simulink model "simulink_scheme_filter"  (R2016b)
settings: Solver=FixedStepAuto  StartTime=0.0  StopTime=20  FixedStep=0.001  RelTol=1e-3
libraries: simulink x1
settings Model: Creator=ram  LastModifiedBy=ram

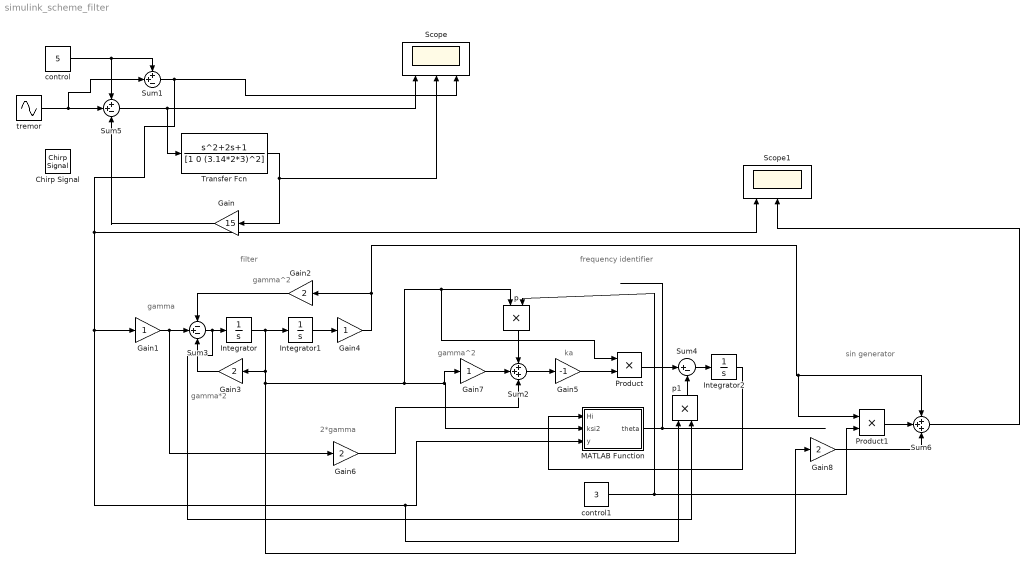
== system simulink_scheme_filter ==
  note: filter
  note: gamma
  note: gamma^2
  note: gamma*2
  note: frequency identifier
  note: ka
  note: 2*gamma
  note: gamma^2
  note: sin generator
  Chirp Signal : simulink/Sources/Chirp Signal  f1=3.14*2*1  T=100  f2=3.14*2*4
  Gain : Gain  Gain=15
  Gain1 : Gain
  Gain{2..3,6,8} (4 alike) : Gain  Gain=2
  Gain4 : Gain
  Gain5 : Gain  Gain=-1
  Gain7 : Gain
  Integrator : Integrator
  Integrator1 : Integrator
  Integrator2 : Integrator
  MATLAB Function : MATLAB Function  TreatAsAtomicUnit=on
  Product : Product
  Product1 : Product
  Scope : Scope  NumInputPorts=3
  Scope1 : Scope  NumInputPorts=3
  Sum1 : Sum  Inputs=++-
  Sum2 : Sum  Inputs=+++
  Sum3 : Sum  Inputs=-+-
  Sum4 : Sum  Inputs=|+-
  Sum5 : Sum  Inputs=++-
  Sum6 : Sum  Inputs=+++
  Transfer Fcn : TransferFcn  Numerator=[1 2 1]  Denominator=[1 0 (3.14*2*3)^2]
  control : Constant  Value=5
  control1 : Constant  Value=3
  p : Product
  p1 : Product
  tremor : Sin  Amplitude=2  Frequency=3.14*2*2  SampleTime=0
  wires:
  control/1 -> Sum5/1, Sum1/1
  Sum5/1 -> Transfer Fcn/1, Scope/1
  Transfer Fcn/1 -> Scope/2, Gain/1
  Gain/1 -> Sum5/3
  Sum3/1 -> p1/2, Integrator/1
  Gain3/1 -> Sum3/3
  Integrator1/1 -> Gain4/1
  Gain1/1 -> Gain6/1, Sum3/2
  Gain2/1 -> Sum3/1
  Sum2/1 -> Gain5/1
  Gain6/1 -> Sum2/3
  tremor/1 -> Sum1/2, Sum5/2
  Gain5/1 -> Product/2
  Gain7/1 -> Sum2/2
  p/1 -> Sum2/1
  Product/1 -> Sum4/1
  p1/1 -> Sum4/2
  Sum1/1 -> Scope/3, p1/1, MATLAB Function/3(y), Gain1/1, Scope1/1
  Sum4/1 -> Integrator2/1
  Integrator2/1 -> MATLAB Function/1(Hi)
  Integrator/1 -> Gain8/1, Product/1, p/1, Gain7/1, MATLAB Function/2(ksi2), Gain3/1, Integrator1/1
  Gain4/1 -> Product1/1, Sum6/1, Gain2/1
  Product1/1 -> Sum6/2
  Sum6/1 -> Scope1/2
  Gain8/1 -> Sum6/3
  MATLAB Function/1(theta) -> ?
  control1/1 -> p/2, Product1/2

== matlab function simulink_scheme_filter/MATLAB Function ==
  data: Hi input; theta output; ksi2 input; y input
function theta = fcn(Hi,ksi2,y)

ka = 1;
gamma = 1;
persistent theta_cup;
if isempty(theta_cup)
    theta_cup = sqrt(3);
    theta = theta_cup;
else
    theta = Hi + theta_cup*ka*gamma^2*ksi2*y;
    theta_cup = theta;
end
end
